simulink model "PlantWTorsionSimulation"  (R2018b)
settings: Solver=VariableStepAuto  StartTime=0.0  StopTime=10.0  RelTol=1e-3
values from neighbouring files (symbols this model uses):
  Delayx = 1    [LinearizePendulumRCSPlant.m]    (also in TestFullStateFeedback.m = Delay(1, i); TestPendulumRCSPlant.m = Delay(1, i); TestPendulumRCSPlantWPsi.m = Delay(1, i); TestQuantizedFullStateFeedback.m = Delay(1, i))
  Delayy = 1    [LinearizePendulumRCSPlant.m]    (also in TestFullStateFeedback.m = Delay(2, i); TestPendulumRCSPlant.m = Delay(2, i); TestPendulumRCSPlantWPsi.m = Delay(2, i); TestQuantizedFullStateFeedback.m = Delay(2, i))
  Fx = 0    [LinearizePendulumRCSPlant.m]    (also in TestFullStateFeedback.m = Fe(1, i); TestPendulumRCSPlant.m = Fe(1, i); TestPendulumRCSPlantWPsi.m = Fe(1, i); TestQuantizedFullStateFeedback.m = Fe(1, i))
  Fy = 0    [LinearizePendulumRCSPlant.m]    (also in TestFullStateFeedback.m = Fe(2, i); TestPendulumRCSPlant.m = Fe(2, i); TestPendulumRCSPlantWPsi.m = Fe(2, i); TestQuantizedFullStateFeedback.m = Fe(2, i))
settings Model: Creator=mendicantbias  LastModifiedBy=mendicantbias

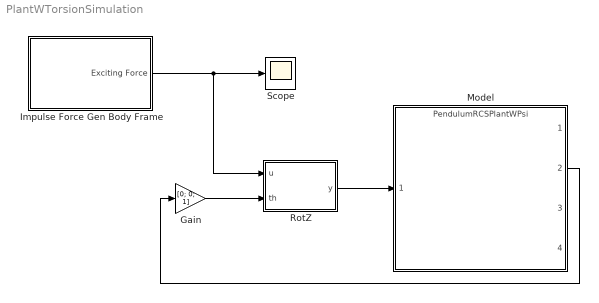
== system PlantWTorsionSimulation ==
  Gain : Gain  Gain=[0; 0; 1]
  Impulse Force Gen Body Frame : Subsystem
  Model : ModelReference  ModelNameDialog=PendulumRCSPlantWPsi  SimulationMode=Normal  ModelReferenceVersion=1.202
  RotZ : MATLAB Function  TreatAsAtomicUnit=on
  Scope : Scope
  wires:
  Impulse Force Gen Body Frame/1("Exciting Force ") -> RotZ/1(u), Scope/1
  Gain/1 -> RotZ/2(th)
  Model/2 -> Gain/1
  RotZ/1(y) -> Model/1

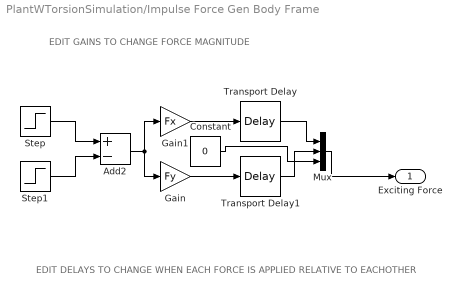
== system PlantWTorsionSimulation/Impulse Force Gen Body Frame ==
  note: EDIT DELAYS TO CHANGE WHEN EACH FORCE IS APPLIED RELATIVE TO EACHOTHER
  note: EDIT GAINS TO CHANGE FORCE MAGNITUDE
  Add2 : Sum  Inputs=+-
  Constant : Constant  Value=0
  Gain : Gain  Gain=Fy
  Gain1 : Gain  Gain=Fx
  Mux : Mux  Inputs=3
  Step : Step  Time=0  SampleTime=0
  Step1 : Step  SampleTime=0
  Transport Delay : TransportDelay  DelayTime=Delayx
  Transport Delay1 : TransportDelay  DelayTime=Delayy
  "Exciting Force " : Outport
  wires:
  Step/1 -> Add2/1
  Step1/1 -> Add2/2
  Add2/1 -> Gain/1, Gain1/1
  Gain1/1 -> Transport Delay/1
  Mux/1 -> "Exciting Force "/1
  Gain/1 -> Transport Delay1/1
  Transport Delay/1 -> Mux/1
  Transport Delay1/1 -> Mux/2
  Constant/1 -> Mux/3

== matlab function PlantWTorsionSimulation/RotZ ==
  data: u input; y output; th input
function y = fcn(u, th)
t = th(3);
Rz = [cos(-t) -sin(-t) 0; sin(-t) cos(-t) 0; 0 0 1];
y = Rz*u;
